simulink model "HeliDraft_26_02_2025"  (R2024b)
settings: Solver=VariableStepAuto  StartTime=0.0  StopTime=10.0  RelTol=1e-3
values from neighbouring files (symbols this model uses):
  R = D/2    (= 2.01773704722)    [untitled.m]
undefined symbols (not defined in the file or in its folder): Afin, AngVel, AngVeltr, BatteryCap, BatteryDischrgRate, Earth, EngPowSL, Ion, Lfin, Lithium, MTOW, Preq2RPM, RPM2Vreq, WGS84
libraries: fl_lib x7, nesl_utility x5, simulink_extras x4, aerolibatmos2 x2, aerolibanimutils x2, aerolibfltsims x2, aerolibtransform2 x1, shared6dof x1, batteryecm_lib x1, spsBatteryLib x1, spsControlledCurrentSourceLib x1, spspowerguiLib x1
(part 1 of 2)
settings Model: Creator=stand-alone1  LastModifiedBy=stand-alone1

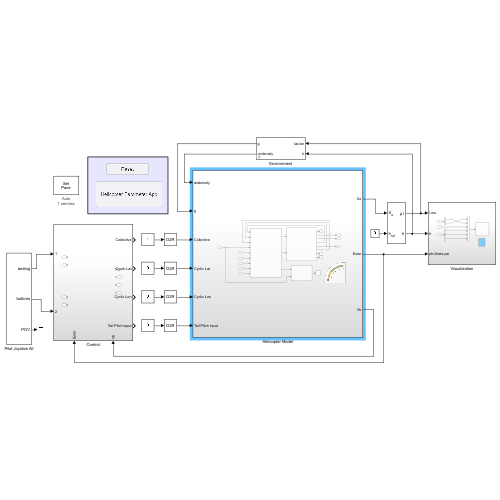
[thumbnail: Simulink's stored preview of the top-level diagram]
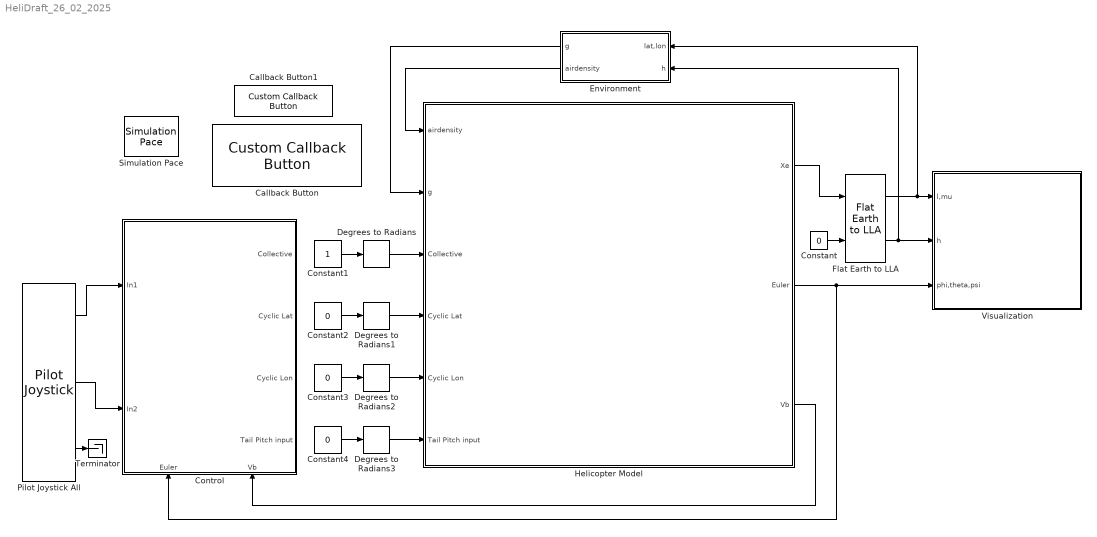
== system HeliDraft_26_02_2025 ==
  Callback Button : CustomCallbackButton  Configuration="{\"components\":[{\"name\":\"BackgroundImageComponent\",\"settings\":{\"image\":{\"size\":[0,0],\"src\":\"default\",\"srcOrientation\":\"Right\"},\"position\":[0,0,1,1]}},{\"name\":\"ButtonStateComponent\",\"settings\":{\"buttonType\":\"momentary\",\"clickFcn\":\"run(\\\"HelicopterParameterEstimation.mlapp\\\");\",\"onValue\":1,\"position\":[0,0,1,1],\"pressDelay\":\"500\",\"pressFcn\":\"\",\"repeatInterval\":\"0\",\"states\":[{\"horizontalAlignment\":\"center\",\"image\":{\"position\":[0,0,1,1],\"size\":[1,1],\"src\":\"default\",\"srcOrientation\":\"Right\"},\"label\":{\"color\":[0.01176470588,0.01176470588,0.01176470588,1],\"icon\":{\"size\":[0,0],\"src\":\"default\",\"srcOrientation\":\"Right\"},\"iconOffset\":0,\"iconPlacement\":\"left\",\"opacity\":1,\"show\":true,\"text\":{\"content\":\"Helicopter Parameter App\",\"font\":\"Helvetica\"}},\"labelOffset\":[0,0],\"verticalAlignment\":\"middle\"},{\"horizontalAlignment\":\"center\",\"image\":{\"position\":[0,0,1,1],\"size\":[1,1],\"src\":\"default\",\"srcOrientation\":\"Right\"},\"label\":{\"color\":[0.01176470588,0.01176470588,0.01176470588,1],\"icon\":{\"size\":[0,0],\"src\":\"default\",\"srcOrientation\":\"Right\"},\"iconOffset\":0,\"iconPlacement\":\"left\",\"opacity\":1,\"show\":true,\"text\":{\"content\":\"Helicopter Parameter App\",\"font\":\"Helvetica\"}},\"labelOffset\":[0,0],\"verticalAlignment\":\"middle\"},{\"horizontalAlignment\":\"center\",\"image\":{\"position\":[0,0,1,1],\"size\":[1,1],\"src\":\"default\",\"srcOrientation\":\"Right\"},\"label\":{\"color\":[0.01176470588,0.01176470588,0.01176470588,1],\"icon\":{\"size\":[0,0],\"src\":\"default\",\"srcOrientation\":\"Right\"},\"iconOffset\":0,\"iconPlacement\":\"left\",\"opacity\":1,\"show\":true,\"text\":{\"content\":\"Helicopter Parameter App\",\"font\":\"Helvetica\"}},\"labelOffset\":[0,0],\"verticalAlignment\":\"middle\"},{\"horizontalAlignment\":\"center\",\"image\":{\"position\":[0,0,1,1],\"size\":[1,1],\"src\":\"default\",\"srcOrientation\":\"Right\"},\"label\":{\"color\":[0.01176470588,0.01176470588,0.01176470588,1],\"icon\":{\"size\":[0,0],\"src\":\"default\",\"srcOrientation\":\"Right\"},\"iconOffset\":0,\"iconPlacement\":\"left\",\"opacity\":1,\"show\":true,\"text\":{\"content\":\"Helicopter Parameter App\",\"font\":\"Helvetica\"}},\"labelOffset\":[0,0],\"verticalAlignment\":\"middle\"}]}},{\"name\":\"ForegroundImageComponent\",\"settings\":{\"image\":{\"size\":[0,0],\"src\":\"default\",\"srcOrientation\":\"Right\"},\"isForeground\":1,\"position\":[0,0,1,1]}}],\"settings\":{\"BindingType\":\"standalone\",\"backgroundColor\":[244,244,244,1],\"backgroundOffset\":0.2,\"backgroundOpacity\":1,\"fixedAspectRatio\":\"off\",\"foregroundColor\":[0.01176470588,0.01176470588,0.01176470588,1],\"migratedFromLegacy\":true,\"useBackgroundColor\":true,\"variant\":\"callback\",\"version\":\"R2023a\"},\"type\":\"Button\"}"  CustomBackgroundColor="{\"color\":[0.9568627451,0.9568627451,0.9568627451],\"show\":true}"
  Callback Button1 : CustomCallbackButton  Configuration="{\"components\":[{\"name\":\"BackgroundImageComponent\",\"settings\":{\"image\":{\"size\":[0,0],\"src\":\"default\",\"srcOrientation\":\"Right\"},\"position\":[0,0,1,1]}},{\"name\":\"ButtonStateComponent\",\"settings\":{\"buttonType\":\"momentary\",\"clickFcn\":\"clc; clear; close all;\",\"onValue\":1,\"position\":[0,0,1,1],\"pressDelay\":\"500\",\"pressFcn\":\"\",\"repeatInterval\":\"0\",\"states\":[{\"horizontalAlignment\":\"center\",\"image\":{\"position\":[0,0,1,1],\"size\":[1,1],\"src\":\"default\",\"srcOrientation\":\"Right\"},\"label\":{\"color\":[0.01176470588,0.01176470588,0.01176470588,1],\"icon\":{\"size\":[0,0],\"src\":\"default\",\"srcOrientation\":\"Right\"},\"iconOffset\":0,\"iconPlacement\":\"left\",\"opacity\":1,\"show\":true,\"text\":{\"content\":\"Reset\",\"font\":\"Helvetica\"}},\"labelOffset\":[0,0],\"verticalAlignment\":\"middle\"},{\"horizontalAlignment\":\"center\",\"image\":{\"position\":[0,0,1,1],\"size\":[1,1],\"src\":\"default\",\"srcOrientation\":\"Right\"},\"label\":{\"color\":[0.01176470588,0.01176470588,0.01176470588,1],\"icon\":{\"size\":[0,0],\"src\":\"default\",\"srcOrientation\":\"Right\"},\"iconOffset\":0,\"iconPlacement\":\"left\",\"opacity\":1,\"show\":true,\"text\":{\"content\":\"Reset\",\"font\":\"Helvetica\"}},\"labelOffset\":[0,0],\"verticalAlignment\":\"middle\"},{\"horizontalAlignment\":\"center\",\"image\":{\"position\":[0,0,1,1],\"size\":[1,1],\"src\":\"default\",\"srcOrientation\":\"Right\"},\"label\":{\"color\":[0.01176470588,0.01176470588,0.01176470588,1],\"icon\":{\"size\":[0,0],\"src\":\"default\",\"srcOrientation\":\"Right\"},\"iconOffset\":0,\"iconPlacement\":\"left\",\"opacity\":1,\"show\":true,\"text\":{\"content\":\"Reset\",\"font\":\"Helvetica\"}},\"labelOffset\":[0,0],\"verticalAlignment\":\"middle\"},{\"horizontalAlignment\":\"center\",\"image\":{\"position\":[0,0,1,1],\"size\":[1,1],\"src\":\"default\",\"srcOrientation\":\"Right\"},\"label\":{\"color\":[0.01176470588,0.01176470588,0.01176470588,1],\"icon\":{\"size\":[0,0],\"src\":\"default\",\"srcOrientation\":\"Right\"},\"iconOffset\":0,\"iconPlacement\":\"left\",\"opacity\":1,\"show\":true,\"text\":{\"content\":\"Reset\",\"font\":\"Helvetica\"}},\"labelOffset\":[0,0],\"verticalAlignment\":\"middle\"}]}},{\"name\":\"ForegroundImageComponent\",\"settings\":{\"image\":{\"size\":[0,0],\"src\":\"default\",\"srcOrientation\":\"Right\"},\"isForeground\":1,\"position\":[0,0,1,1]}}],\"settings\":{\"BindingType\":\"standalone\",\"backgroundColor\":[244,244,244,1],\"backgroundOffset\":0.2,\"backgroundOpacity\":1,\"fixedAspectRatio\":\"off\",\"foregroundColor\":[0.01176470588,0.01176470588,0.01176470588,1],\"migratedFromLegacy\":true,\"useBackgroundColor\":true,\"variant\":\"callback\",\"version\":\"R2023a\"},\"type\":\"Button\"}"  CustomBackgroundColor="{\"color\":[0.9568627451,0.9568627451,0.9568627451],\"show\":true}"
  Constant{,2..4} (4 alike) : Constant  Value=0
  Constant1 : Constant
  Control : Subsystem
      settings: PortSchema="{\"entries\":[{\"content\":{\"sides\":[{\"content\":{\"connectorIds\":[\"In1\",\"In2\"]},\"type\":\"ConnectorPlacement.EquallySpacedRectSide\",\"uuid\":\"528401e7-0fef-44be-ba63-acf96d247fb7\"},{\"content\":{\"connectorIds\":[\"Out1\",\"Out2\",\"Out3\",\"Out4\"],\"side\":\"RIGHT\"},\"type\":\"ConnectorPlacement.EquallySpacedRectSide\",\"uuid\":\"314663aa-6cd9-4175-a49a-1575f8a7b87b\"},{\"content\":{\"side\":\"TOP\"},\"type\":\"ConnectorPlacement.EquallySpacedRectSide\",\"uuid\":\"d6c3b2b9-365b-49fe-86cc-8f0c15878230\"},{\"content\":{\"connectorIds\":[\"In3\",\"In4\"],\"side\":\"BOTTOM\"},\"type\":\"ConnectorPlacement.EquallySpacedRectSide\",\"uuid\":\"be77d0ba-d3ca-47ac-ab5e-0cf95d8527f7\"}]},\"type\":\"ConnectorPlacement.EquallySpacedConnector\",\"uuid\":\"719848b2-01be-4853-b472-0e21e9b8be5c\"}],\"packageUris\":[\"http://schema.mathworks.com/mf0/Connector/R2020b\"],\"version\":\"1.0\"}"
  Degrees to Radians{,1..3} (4 alike) : simulink_extras/Transformations/Degrees to Radians
  Environment : Subsystem  mask{atmomodel=ISA, consg=on, Parameter3=on}
      mask prompts: atmomodel "Atmosphere Model"; consg "Constant g (Gravitational Acceleration)"; Parameter3 "On/Off"
      mask DialogControl a Prompt: Environment
      mask DialogControl b Prompt: Wind simulation, atmosphere properties and gravity model
      mask DialogControl Container4 Prompt: Environment
      mask DialogControl Container5 Prompt: Wind
  Flat Earth to LLA : aerolibtransform2/Flat Earth to LLA  units=Metric (MKS)  ptype=Earth (WGS84)  F=1/298.257223563  R=6378137  refPosPort=off  LL0=[0 10]  psi=0
  Helicopter Model : Subsystem
  Pilot Joystick All : aerolibanimutils/Pilot Joystick  JoystickID=Joystick1  OutputConfiguration=AllOutputs  SampleTime=1/30
      settings: LibrarySourceBlock=aerolibanimutils/Pilot Joystick All
  Simulation Pace : aerolibanimutils/Simulation Pace  SimulationPace=1  SleepMode=Auto  OutputPaceError=off  SampleTime=1/30
  Terminator : Terminator
  Visualization : Subsystem
  wires:
  Constant/1 -> Flat Earth to LLA/2
  Flat Earth to LLA/1 -> Environment/1(lat,lon), Visualization/1(l,mu)
  Flat Earth to LLA/2 -> Environment/2(h), Visualization/2(h)
  Pilot Joystick All/1 -> Control/1(In1)
  Pilot Joystick All/2 -> Control/2(In2)
  Environment/1(g) -> Helicopter Model/2(g)
  Environment/2(airdensity) -> Helicopter Model/1(airdensity)
  Helicopter Model/1(Xe) -> Flat Earth to LLA/1
  Helicopter Model/2(Euler) -> Visualization/3(phi,theta,psi), Control/3(Euler)
  Pilot Joystick All/3 -> Terminator/1
  Helicopter Model/3(Vb) -> Control/4(Vb)
  Constant1/1 -> Degrees to Radians/1
  Constant2/1 -> Degrees to Radians1/1
  Constant3/1 -> Degrees to Radians2/1
  Constant4/1 -> Degrees to Radians3/1
  Degrees to Radians/1 -> Helicopter Model/3(Collective)
  Degrees to Radians1/1 -> Helicopter Model/4(Cyclic Lat)
  Degrees to Radians2/1 -> Helicopter Model/5(Cyclic Lon)
  Degrees to Radians3/1 -> Helicopter Model/6(Tail Pitch input)

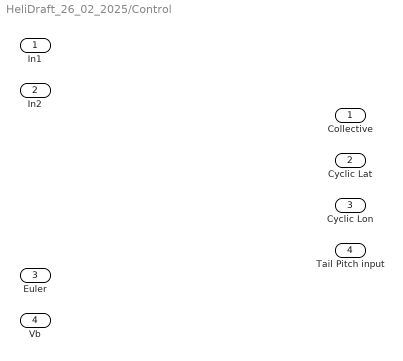
== system HeliDraft_26_02_2025/Control ==
  In1 : Inport
  In2 : Inport  Port=2
  Euler : Inport  Port=3
  Vb : Inport  Port=4
  Collective : Outport
  Cyclic Lat : Outport  Port=2
  Cyclic Lon : Outport  Port=3
  Tail Pitch input : Outport  Port=4

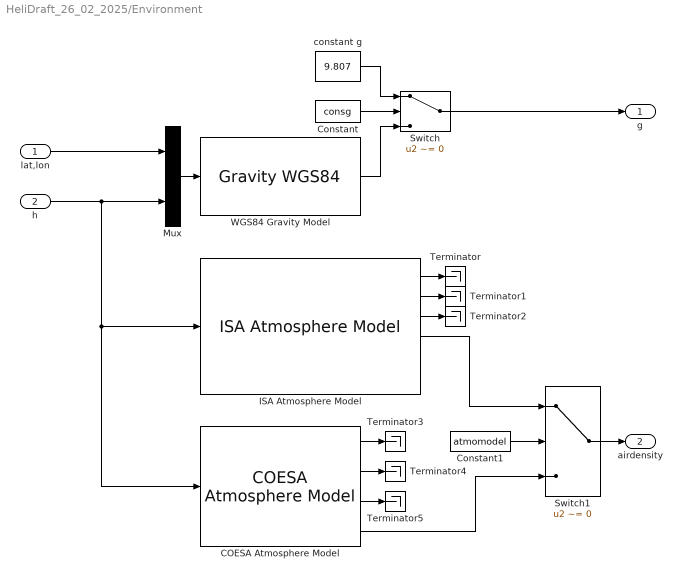
== system HeliDraft_26_02_2025/Environment ==
  lat,lon : Inport
  h : Inport  Port=2
  COESA Atmosphere Model : aerolibatmos2/COESA Atmosphere Model  units=Metric (MKS)  spec=1976 COESA-extended U.S. Standard Atmosphere  model=Profile  profile_var=High temperature  profile_percent=1%  profile_alt=5 km (16404 ft)  envelope_var=High temperature  envelope_percent=1%  action=Warning
  Constant : Constant  Value=consg
  Constant1 : Constant  Value=atmomodel
  ISA Atmosphere Model : aerolibatmos2/ISA Atmosphere Model  useExtended=off  action=Warning  custom=off  viscosityOut=on  g=9.80665  gamma=1.4  R=287.0531  L=0.0065  h_trop=11000  h_strat=20000  rho0=1.225  P0=101325  T0=288.15  h0=0  S=110.4  Tref=273.15  muref=1.716e-5
  Mux : Mux  Inputs=2
  Switch : Switch  Criteria=u2 ~= 0  SaturateOnIntegerOverflow=off  InputSameDT=off
  Switch1 : Switch  Criteria=u2 ~= 0  SaturateOnIntegerOverflow=off  InputSameDT=off
  Terminator{,1..5} (6 alike) : Terminator
  "WGS84 Gravity Model  " : GravityWGS84
  constant g : Constant  Value=9.807
  g : Outport
  airdensity : Outport  Port=2
  wires:
  lat,lon/1 -> Mux/1
  Constant/1 -> Switch/2
  constant g/1 -> Switch/1
  "WGS84 Gravity Model  "/1 -> Switch/3
  Switch/1 -> g/1
  Mux/1 -> "WGS84 Gravity Model  "/1
  h/1 -> COESA Atmosphere Model/1, ISA Atmosphere Model/1, Mux/2
  Switch1/1 -> airdensity/1
  ISA Atmosphere Model/1 -> Terminator/1
  ISA Atmosphere Model/2 -> Terminator1/1
  ISA Atmosphere Model/3 -> Terminator2/1
  COESA Atmosphere Model/2 -> Terminator4/1
  COESA Atmosphere Model/1 -> Terminator3/1
  COESA Atmosphere Model/3 -> Terminator5/1
  ISA Atmosphere Model/4 -> Switch1/1
  COESA Atmosphere Model/4 -> Switch1/3
  Constant1/1 -> Switch1/2

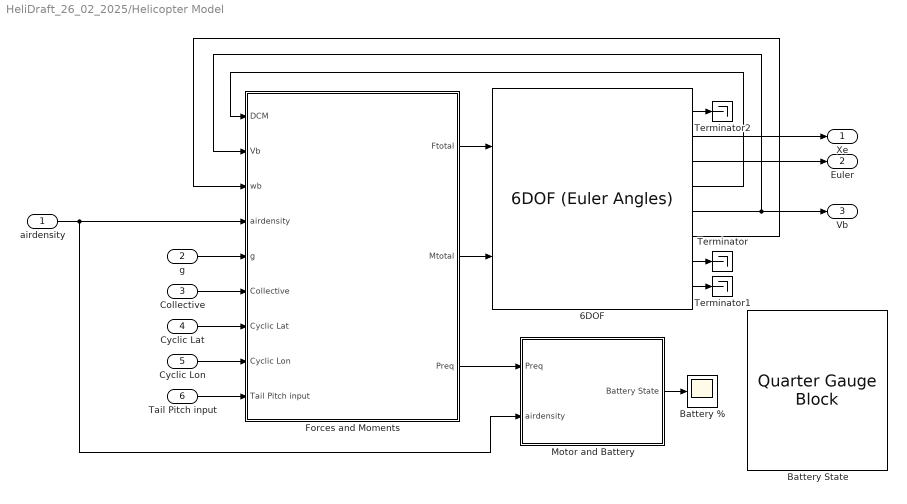
== system HeliDraft_26_02_2025/Helicopter Model ==
  airdensity : Inport
  g : Inport  Port=2
  Collective : Inport  Port=3
  Cyclic Lat : Inport  Port=4
  Cyclic Lon : Inport  Port=5
  Tail Pitch input : Inport  Port=6
  6DOF : shared6dof/6DOF (Euler Angles)  units=Metric (MKS)  mtype=Fixed  rep=Euler Angles  xme_0=[0 0 0]  Vm_0=[0 0 0]  eul_0=[0 0 0]  pm_0=[0 0 0]  mass_0=MTOW  mass_e=0.5  mass_f=2.0  inertia=eye(3)  inertia_e=eye(3)  inertia_f=2*eye(3)  k_quat=1.0  vre_flag=off  abi_flag=off  aMode=0  xme_statename=''  Vm_statename=''  eul_statename=''  quat_statename=''  pm_statename=''  mass_statename=''
  Battery % : Scope
  Battery State : QuarterGaugeBlock  LabelPosition=Hide
  Forces and Moments : Subsystem
  Motor and Battery : Subsystem
  Terminator : Terminator
  Terminator1 : Terminator
  Terminator2 : Terminator
  Xe : Outport
  Euler : Outport  Port=2
  Vb : Outport  Port=3
  wires:
  6DOF/1 -> Terminator2/1
  6DOF/8 -> Terminator1/1
  Forces and Moments/1(Ftotal) -> 6DOF/1
  Forces and Moments/2(Mtotal) -> 6DOF/2
  6DOF/6 -> Forces and Moments/3(wb)
  6DOF/4 -> Forces and Moments/1(DCM)
  6DOF/7 -> Terminator/1
  6DOF/5 -> Vb/1, Forces and Moments/2(Vb)
  Cyclic Lat/1 -> Forces and Moments/7(Cyclic Lat)
  Collective/1 -> Forces and Moments/6(Collective)
  6DOF/3 -> Euler/1
  Tail Pitch input/1 -> Forces and Moments/9(Tail Pitch input)
  Cyclic Lon/1 -> Forces and Moments/8(Cyclic Lon)
  airdensity/1 -> Forces and Moments/4(airdensity), Motor and Battery/2(airdensity)
  g/1 -> Forces and Moments/5(g)
  6DOF/2 -> Xe/1
  Forces and Moments/3(Preq) -> Motor and Battery/1(Preq)
  Motor and Battery/1(Battery State) -> Battery %/1

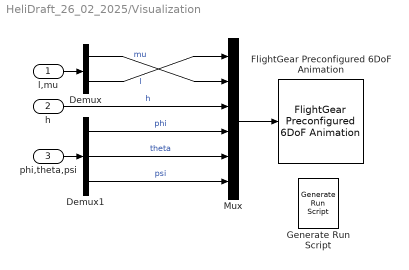
== system HeliDraft_26_02_2025/Visualization ==
  l,mu : Inport
  h : Inport  Port=2
  phi,theta,psi : Inport  Port=3
  Demux : Demux  Outputs=2
  Demux1 : Demux  Outputs=3
  "FlightGear Preconfigured 6DoF Animation " : aerolibfltsims/FlightGear Preconfigured 6DoF Animation  xFlightGearVersion=v2019.1  DestinationIpAddress=127.0.0.1  DestinationPort=5502  SampleTime=1/30  packetVersion=24
  "Generate Run Script " : aerolibfltsims/Generate Run Script  Architecture=Default  dataFlow=Send  GeometryModelName=HL20  AirportId=KSFO  RunwayId=10L  InitialAltitude=7224  InitialHeading=113  OffsetDistance=4.72  OffsetAzimuth=0  InstallScenery=off  DisableShaders=off  OriginAddress=127.0.0.1  DestinationPort=5502  OriginPort=5505  LocalAddress=127.0.0.1  OutputFileName=runfg.bat  FlightGearBaseDirectory=C:\Program Files\FlightGear
  Mux : Mux  Inputs=6
  wires:
  l,mu/1 -> Demux/1
  Demux/2 -> Mux/1  "l"
  Demux/1 -> Mux/2  "mu"
  Mux/1 -> "FlightGear Preconfigured 6DoF Animation "/1
  h/1 -> Mux/3  "h"
  Demux1/1 -> Mux/4  "phi"
  Demux1/2 -> Mux/5  "theta"
  Demux1/3 -> Mux/6  "psi"
  phi,theta,psi/1 -> Demux1/1

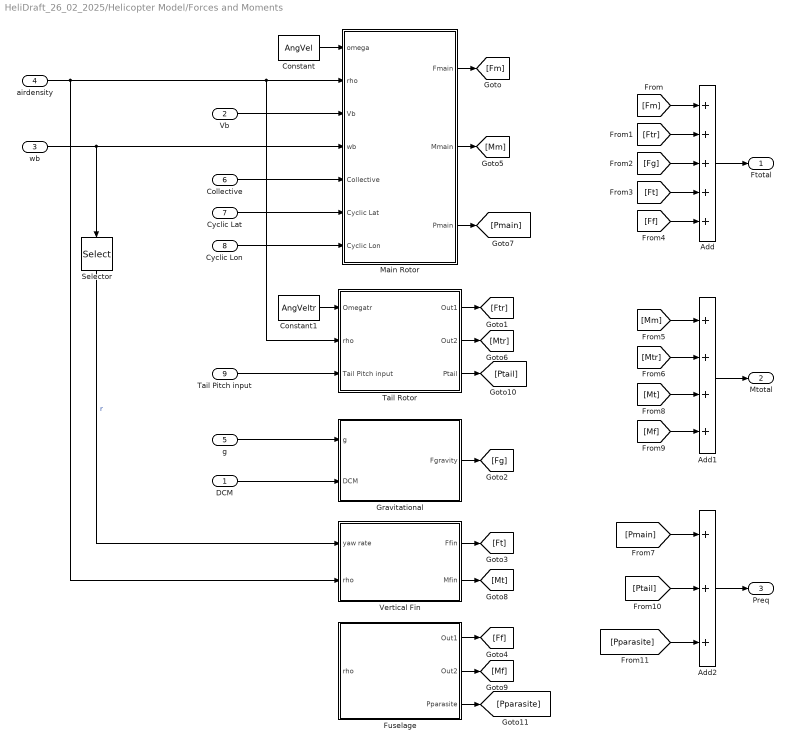
== system HeliDraft_26_02_2025/Helicopter Model/Forces and Moments ==
  DCM : Inport
  Vb : Inport  Port=2
  wb : Inport  Port=3
  airdensity : Inport  Port=4
  g : Inport  Port=5
  Collective : Inport  Port=6
  Cyclic Lat : Inport  Port=7
  Cyclic Lon : Inport  Port=8
  Tail Pitch input : Inport  Port=9
  Add : Sum  Inputs=+++++
  Add1 : Sum  Inputs=++++
  Add2 : Sum  Inputs=+++
  Constant : Constant  Value=AngVel
  Constant1 : Constant  Value=AngVeltr
  Fuselage : Subsystem
  Gravitational : Subsystem
  Main Rotor : Subsystem
  Selector : Selector  InputPortWidth=3  IndexOptions=Index vector (dialog)  Indices=[3]  OutputSizes=1
  Tail Rotor : Subsystem
  Vertical Fin : Subsystem
  Ftotal : Outport
  Mtotal : Outport  Port=2
  Preq : Outport  Port=3
  wires:
  Add/1 -> Ftotal/1
  Add1/1 -> Mtotal/1
  Main Rotor/1(Fmain) -> [Fm]
  Tail Rotor/1(Out1) -> [Ftr]
  Gravitational/1(Fgravity) -> [Fg]
  Vertical Fin/1(Ffin) -> [Ft]
  Fuselage/1(Out1) -> [Ff]
  [Fm] -> Add/1
  [Ftr] -> Add/2
  [Fg] -> Add/3
  [Ft] -> Add/4
  [Ff] -> Add/5
  Main Rotor/2(Mmain) -> [Mm]
  Tail Rotor/2(Out2) -> [Mtr]
  Vertical Fin/2(Mfin) -> [Mt]
  Fuselage/2(Out2) -> [Mf]
  [Mm] -> Add1/1
  [Mtr] -> Add1/2
  [Mf] -> Add1/4
  [Mt] -> Add1/3
  Constant/1 -> Main Rotor/1(omega)
  Constant1/1 -> Tail Rotor/1(Omegatr)
  airdensity/1 -> Vertical Fin/2(rho), Tail Rotor/2(rho), Main Rotor/2(rho)
  g/1 -> Gravitational/1(g)
  DCM/1 -> Gravitational/2(DCM)
  Collective/1 -> Main Rotor/5(Collective)
  Tail Pitch input/1 -> Tail Rotor/3(Tail Pitch input)
  Cyclic Lat/1 -> Main Rotor/6(Cyclic Lat)
  Cyclic Lon/1 -> Main Rotor/7(Cyclic Lon)
  wb/1 -> Selector/1, Main Rotor/4(wb)
  Vb/1 -> Main Rotor/3(Vb)
  Add2/1 -> Preq/1
  Main Rotor/3(Pmain) -> [Pmain]
  Tail Rotor/3(Ptail) -> [Ptail]
  Fuselage/3(Pparasite) -> [Pparasite]
  [Pmain] -> Add2/1
  [Ptail] -> Add2/2
  [Pparasite] -> Add2/3
  Selector/1 -> Vertical Fin/1(yaw rate)  "r"

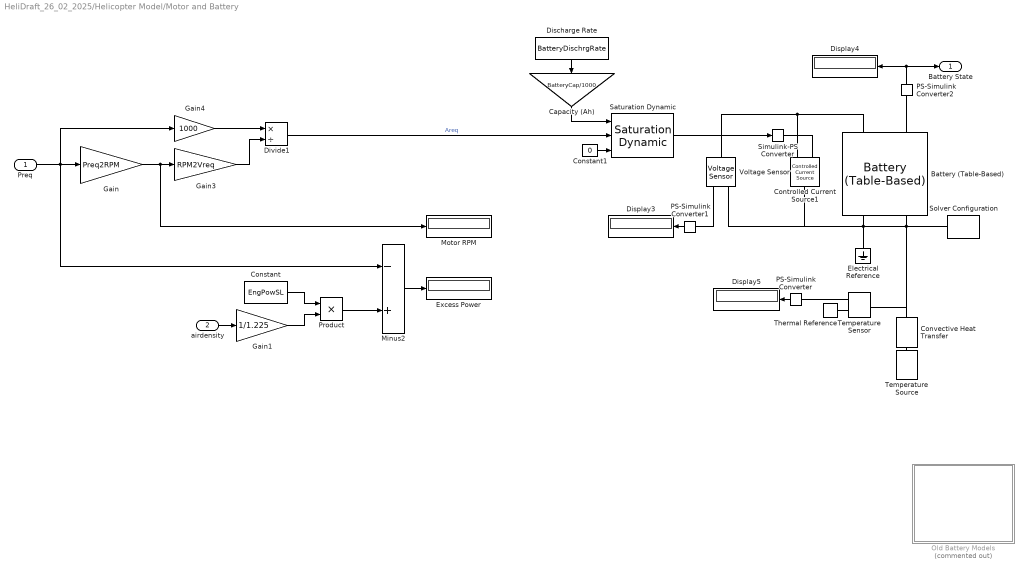
== system HeliDraft_26_02_2025/Helicopter Model/Motor and Battery ==
  Preq : Inport
  airdensity : Inport  Port=2
  Battery (Table-Based) : batteryecm_lib/Battery (Table-Based)  PartSpecification="{\"DatasetId\":\"Valence|U27_36XP|simscape.battery.batteryTableBased\",\"DisplayName\":\"Valence:U27_36XP\"}"  SOC_vec=[0 0.01 0.02 0.03 0.04 0.05 0.06 0.07 0.08 0.09 0.1 0.11 0.12 0.13 0.14 0.15 0.16 0.17 0.18 0.19 0.2 0.21 0.22 0.23 0.24 0.25 0.26 0.27 0.28 0.29 0.3 0.31 0.32 0.33 0.34 0.35 0.36 0.37 0.38 0.39 0.4 0.41 0.42 0.43 0.44 0.45 0.46 0.47 0.48 0.49 0.5 0.51 0.52 0.53 0.54 0.55 0.56 0.57 0.58 0.59 0.6 0.61 0.62 0.63 0.64 0.65 0.66 0.67 0.68 0.69 0.7 0.71 0.72 0.73 0.74 0.75 0.76 0.77 0.78 0.79 0.8 0.81 0.82 0.83 0.84 0.85 0.86 0.87 0.88 0.89 0.9 0.91 0.92 0.93 0.94 0.95 0.96 0.97 0.98 0.99 1] % Datasheet derived  T_dependence=simscape.enum.tablebattery.temperature_dependence.yes  prm_dir=simscape.enum.tablebattery.prm_dir.noCurrentDirectionality  T_vec=[-10 0 10 20 23 30 40 50] % Datasheet derived degC  V0_mat=[35.84591 35.84591 35.84591 35.84591 35.84591 35.84591 35.84591 35.84591;36.10202 36.10202 36.10202 36.10202 36.10202 36.10202 36.10202 36.10202;36.35814 36.35814 36.35814 36.35814 36.35814 36.35814 36.35814 36.35814;36.61425 36.61425 36.61425 36.61425 36.61425 36.61425 36.61425 36.61425;36.87037 36.87037 36.87037 36.87037 36.87037 36.87037 36.87037 36.87037;37.12649 37.12649 37.12649 37.12649 37.12649 37.12649 37.12649 37.12649;37.3826 37.3826 37.3826 37.3826 37.3826 37.3826 37.3826 37.3826;37.63872 37.63872 37.63872 37.63872 37.63872 37.63872 37.63872 37.63872;37.89483 37.89483 37.89483 37.89483 37.89483 37.89483 37.89483 37.89483;38.09951 38.09951 38.09951 38.09951 38.09951 38.09951 38.09951 38.09951;38.20904 38.20904 38.20904 38.20904 38.20904 38.20904 38.20904 38.20904;38.28916 38.28916 38.28916 38.28916 38.28916 38.28916 38.28916 38.28916;38.37306 38.37306 38.37306 38.37306 38.37306 38.37306 38.37306 38.37306;38.42308 38.42308 38.42308 38.42308 38.42308 38.42308 38.42308 38.42308;38.45482 38.45482 38.45482 38.45482 38.45482 38.45482 38.45482 38.45482;38.47744 38.47744 38.47744 38.47744 38.47744 38.47744 38.47744 38.47744;38.49779 38.49779 38.49779 38.49779 38.49779 38.49779 38.49779 38.49779;38.54815 38.54815 38.54815 38.54815 38.54815 38.54815 38.54815 38.54815;38.5883 38.5883 38.5883 38.5883 38.5883 38.5883 38.5883 38.5883;38.63829 38.63829 38.63829 38.63829 38.63829 38.63829 38.63829 38.63829;38.68732 38.68732 38.68732 38.68732 38.68732 38.68732 38.68732 38.68732;38.72975 38.72975 38.72975 38.72975 38.72975 38.72975 38.72975 38.72975;38.77111 38.77111 38.77111 38.77111 38.77111 38.77111 38.77111 38.77111;38.80795 38.80795 38.80795 38.80795 38.80795 38.80795 38.80795 38.80795;38.83724 38.83724 38.83724 38.83724 38.83724 38.83724 38.83724 38.83724;38.8617 38.8617 38.8617 38.8617 38.8617 38.8617 38.8617 38.8617;38.89023 38.89023 38.89023 38.89023 38.89023 38.89023 38.89023 38.89023;38.9273 38.9273 38.9273 38.9273 38.9273 38.9273 38.9273 38.9273;38.96054 38.96054 38.96054 38.96054 38.96054 38.96054 38.96054 38.96054;38.98786 38.98786 38.98786 38.98786 38.98786 38.98786 38.98786 38.98786;39.01519 39.01519 39.01519 39.01519 39.01519 39.01519 39.01519 39.01519;39.03864 39.03864 39.03864 39.03864 39.03864 39.03864 39.03864 39.03864;39.06385 39.06385 39.06385 39.06385 39.06385 39.06385 39.06385 39.06385;39.08223 39.08223 39.08223 39.08223 39.08223 39.08223 39.08223 39.08223;39.1006 39.1006 39.1006 39.1006 39.1006 39.1006 39.1006 39.1006;39.11898 39.11898 39.11898 39.11898 39.11898 39.11898 39.11898 39.11898;39.13735 39.13735 39.13735 39.13735 39.13735 39.13735 39.13735 39.13735;39.15508 39.15508 39.15508 39.15508 39.15508 39.15508 39.15508 39.15508;39.16412 39.16412 39.16412 39.16412 39.16412 39.16412 39.16412 39.16412;39.17437 39.17437 39.17437 39.17437 39.17437 39.17437 39.17437 39.17437;39.18528 39.18528 39.18528 39.18528 39.18528 39.18528 39.18528 39.18528;39.19619 39.19619 39.19619 39.19619 39.19619 39.19619 39.19619 39.19619;39.20709 39.20709 39.20709 39.20709 39.20709 39.20709 39.20709 39.20709;39.21696 39.21696 39.21696 39.21696 39.21696 39.21696 39.21696 39.21696;39.22232 39.22232 39.22232 39.22232 39.22232 39.22232 39.22232 39.22232;39.22753 39.22753 39.22753 39.22753 39.22753 39.22753 39.22753 39.22753;39.23277 39.23277 39.23277 39.23277 39.23277 39.23277 39.23277 39.23277;39.23672 39.23672 39.23672 39.23672 39.23672 39.23672 39.23672 39.23672;39.23942 39.23942 39.23942 39.23942 39.23942 39.23942 39.23942 39.23942;39.24211 39.24211 39.24211 39.24211 39.24211 39.24211 39.24211 39.24211;39.24481 39.24481 39.24481 39.24481 39.24481 39.24481 39.24481 39.24481;39.24786 39.24786 39.24786 39.24786 39.24786 39.24786 39.24786 39.24786;39.25094 39.25094 39.25094 39.25094 39.25094 39.25094 39.25094 39.25094;39.2539 39.2539 39.2539 39.2539 39.2539 39.2539 39.2539 39.2539;39.25686 39.25686 39.25686 39.25686 39.25686 39.25686 39.25686 39.25686;39.26099 39.26099 39.26099 39.26099 39.26099 39.26099 39.26099 39.26099;39.26708 ...(+3199 chars)] % Datasheet derived V  V0_vec=[35.84591 36.10202 36.35814 36.61425 36.87037 37.12649 37.3826 37.63872 37.89483 38.09951 38.20904 38.28916 38.37306 38.42308 38.45482 38.47744 38.49779 38.54815 38.5883 38.63829 38.68732 38.72975 38.77111 38.80795 38.83724 38.8617 38.89023 38.9273 38.96054 38.98786 39.01519 39.03864 39.06385 39.08223 39.1006 39.11898 39.13735 39.15508 39.16412 39.17437 39.18528 39.19619 39.20709 39.21696 39.22232 39.22753 39.23277 39.23672 39.23942 39.24211 39.24481 39.24786 39.25094 39.2539 39.25686 39.26099 39.26708 39.27551 39.28394 39.29233 39.30067 39.31557 39.33487 39.35402 39.37113 39.38825 39.40815 39.43406 39.46187 39.48968 39.51913 39.55031 39.5817 39.60619 39.62271 39.63907 39.65521 39.67134 39.68137 39.69071 39.70005 39.7052 39.70868 39.70916 39.70862 39.70807 39.70752 39.71037 39.72142 39.72908 39.73651 39.73911 39.73577 39.72919 39.73278 39.7392 39.74638 39.75462 39.8136 40.01141 40.30627] % Datasheet derived V  V_range=[27 Inf] % Datasheet derived V  R0_mat=[0.9112 0.73319 0.55116 0.3909 0.47635 0.31145 0.24894 0.23351;0.9112 0.79214 0.50936 0.32708 0.41138 0.21289 0.15029 0.11642;0.9112 0.75838 0.46755 0.26325 0.35007 0.14203 0.09214 0.07324;0.9112 0.72463 0.42575 0.19942 0.29417 0.09634 0.05758 0.04021;0.9112 0.69087 0.38395 0.15149 0.24882 0.06764 0.03364 0.02182;0.9112 0.65711 0.34215 0.11725 0.2142 0.04885 0.01957 0.00983;0.9112 0.62335 0.30035 0.09581 0.18886 0.03484 0.01134 0.00372;0.88245 0.58959 0.25855 0.08105 0.17031 0.02886 0.01013 0.00445;0.85369 0.55583 0.22327 0.07125 0.1569 0.02915 0.01483 0.00976;0.82493 0.52207 0.19506 0.06386 0.14398 0.03152 0.0196 0.01392;0.79618 0.48831 0.16793 0.05824 0.13028 0.031 0.02172 0.01735;0.76742 0.45455 0.14437 0.05231 0.11716 0.03152 0.02306 0.0196;0.73866 0.42079 0.12447 0.04884 0.10632 0.03219 0.02454 0.02192;0.70991 0.38703 0.1096 0.04638 0.09512 0.03151 0.02458 0.0216;0.68115 0.35327 0.09525 0.04318 0.08414 0.02987 0.02387 0.02054;0.65239 0.31952 0.08121 0.03996 0.07347 0.02787 0.02226 0.01912;0.62364 0.27915 0.07388 0.03692 0.06467 0.02578 0.02045 0.01757;0.59488 0.24506 0.06774 0.03508 0.05964 0.02492 0.01984 0.01722;0.56612 0.21466 0.06284 0.03384 0.05477 0.02422 0.01882 0.01646;0.53737 0.18917 0.06009 0.03346 0.05154 0.02391 0.0187 0.0161;0.50861 0.16681 0.05729 0.03301 0.04841 0.02357 0.0188 0.0157;0.47986 0.14646 0.05423 0.03228 0.04625 0.02296 0.01864 0.01586;0.4511 0.13143 0.05231 0.0315 0.04448 0.02305 0.01844 0.01609;0.42234 0.11995 0.05123 0.03055 0.04297 0.02298 0.01851 0.01613;0.39359 0.10903 0.04985 0.03032 0.04112 0.02261 0.01828 0.01587;0.36483 0.09944 0.04828 0.02989 0.03908 0.02204 0.01786 0.01541;0.33607 0.09353 0.04687 0.02963 0.0378 0.02164 0.01762 0.01512;0.30291 0.08834 0.04648 0.02972 0.03771 0.02158 0.01779 0.01527;0.27067 0.08411 0.04619 0.02964 0.03746 0.0219 0.0178 0.01525;0.24264 0.08054 0.04566 0.02987 0.03699 0.02206 0.01758 0.015;0.21621 0.07803 0.04513 0.03012 0.03652 0.02222 0.01736 0.01476;0.19063 0.07544 0.04456 0.03022 0.03598 0.02223 0.01698 0.01435;0.17492 0.07417 0.04451 0.03039 0.03587 0.0223 0.01675 0.01402;0.15924 0.07263 0.04418 0.03029 0.03552 0.0221 0.01669 0.01376;0.14506 0.07109 0.04385 0.03019 0.03517 0.0219 0.01663 0.01361;0.13357 0.06955 0.04352 0.03009 0.03481 0.0217 0.01658 0.01346;0.12461 0.0686 0.04319 0.02998 0.03446 0.0215 0.01652 0.01331;0.11872 0.06771 0.04286 0.02995 0.03417 0.02128 0.01643 0.01313;0.11354 0.06648 0.04251 0.02967 0.03358 0.02084 0.016 0.01261;0.10849 0.0653 0.0422 0.02943 0.03336 0.02078 0.01562 0.01213;0.10559 0.06415 0.04193 0.02923 0.03321 0.02075 0.01526 0.01187;0.10269 0.06364 0.04165 0.02902 0.03305 0.02071 0.01515 0.01197;0.09978 0.06339 0.04137 0.02881 0.0329 0.02068 0.01521 0.01208;0.09733 0.06309 0.04105 0.02856 0.0327 0.0206 0.01523 0.01214;0.09518 0.06261 0.0406 0.02813 0.03227 0.02035 0.01507 0.01203;0.09303 0.06213 0.04031 0.0277 0.03186 0.02009 0.01491 0.01191;0.0912 0.06165 0.04003 0.02736 0.03148 0.01983 0.01474 0.01179;0.08999 0.06112 0.0397 0.02706 0.03105 0.01963 0.01452 0.01161;0.08874 0.06053 0.03932 0.02671 0.03058 0.0194 0.01426 0.01139;0.08749 0.05993 0.03893 0.02636 0.03011 0.01916 0.01399 0.01119;0.08652 0.05934 0.03855 0.02601 0.02964 0.01893 0.01372 0.01104;0.08605 0.05876 0.03818 0.02568 0.02918 0.01872 0.01346 0.01091;0.08557 0.05819 0.03788 0.02534 0.02875 0.0185 0.0132 0.01078;0.0851 0.0576 0.03759 0.025 0.02834 0.01828 0.01294 0.01065;0.08479 0.05702 0.0373 0.02466 0.02792 0.01806 0.01268 0.01051;0.08459 0.05663 0.03706 0.0244 0.02762 0.01789 0.01247 0.01042;0.08446 0.0566 0.0369 0.02423 0.02745 0.01779 0.01233 0.01038;0.08442 0.05667 0.03684 0.02414 0.02737 0.01779 0.01229 0.01018;0.08439 0.05674 0.03677 0.02406 0.02729 0.01777 0.01225 0.00997;0.08436 0.05681 0.0367 0.02397 0.02722 0.01767 0.01221 0.00977;0.08463 0.05687 0.03669 0.02389 0.02715 0.01757 0.01218 0.00956;0.08516 0.0572 0.03698 0.02406 0.0274 0.01773 0.0124 0.00962;0.08586 0.0577 0.03744 0.02442 0.02786 0.01806 0.0128 0.00985;0.08657 0.05819 0.0379 ...(+2382 chars)] % Datasheet derived Ohm  R0_vec=[0.47635 0.41138 0.35007 0.29417 0.24882 0.2142 0.18886 0.17031 0.1569 0.14398 0.13028 0.11716 0.10632 0.09512 0.08414 0.07347 0.06467 0.05964 0.05477 0.05154 0.04841 0.04625 0.04448 0.04297 0.04112 0.03908 0.0378 0.03771 0.03746 0.03699 0.03652 0.03598 0.03587 0.03552 0.03517 0.03481 0.03446 0.03417 0.03358 0.03336 0.03321 0.03305 0.0329 0.0327 0.03227 0.03186 0.03148 0.03105 0.03058 0.03011 0.02964 0.02918 0.02875 0.02834 0.02792 0.02762 0.02745 0.02737 0.02729 0.02722 0.02715 0.0274 0.02786 0.0283 0.02854 0.02877 0.02906 0.02956 0.03013 0.0307 0.03135 0.03204 0.03271 0.03308 0.03307 0.03314 0.03323 0.03332 0.03312 0.03288 0.03264 0.03224 0.03172 0.03113 0.03057 0.03001 0.02945 0.02905 0.02924 0.0293 0.02938 0.02923 0.02879 0.02803 0.02792 0.02793 0.02786 0.02652 0.02587 0.02701 0.00941] % Datasheet derived Ohm  R0_dis_mat=[.0117, .0085, .009; .011, .0085, .009; .0114, .0087, .0092; .0107, .0082, .0088; .0107, .0083, .0091; .0113, .0085, .0089; .0116, .0085, .0089] % Parameter not set Ohm  R0_dis_vec=[.0085, .0085, .0087, .0082, .0083, .0085, .0085] % Parameter not set Ohm  R0_ch_mat=[.0117, .0085, .009; .011, .0085, .009; .0114, .0087, .0092; .0107, .0082, .0088; .0107, .0083, .0091; .0113, .0085, .0089; .0116, .0085, .0089] % Parameter not set Ohm  R0_ch_vec=[.0085, .0085, .0087, .0082, .0083, .0085, .0085] % Parameter not set Ohm  AH=50.41 % Datasheet derived hr*A  prm_leak=simscape.enum.tablebattery.prm_leak.disabled  Rleak_vec=[8000, 7000, 6000] % Parameter not set Ohm  Rleak=7e3 % Parameter not set Ohm  extrapolation_option=simscape.enum.extrapolation.nearest  SOC_port=simscape.enum.tablebattery.enable.yes  prm_dyn=simscape.enum.tablebattery.prm_dyn.off  R1_mat=[.0109, .0029, .0013; .0069, .0024, .0012; .0047, .0026, .0013; .0034, .0016, .001; .0033, .0023, .0014; .0033, .0018, .0011; .0028, .0017, .0011] % Parameter not set Ohm  R1_vec=[.0029, .0024, .0026, .0016, .0023, .0018, .0017] % Parameter not set Ohm  tau1_mat=[20, 36, 39; 31, 45, 39; 109, 105, 61; 36, 29, 26; 59, 77, 67; 40, 33, 29; 25, 39, 33] % Parameter not set s  tau1_vec=[36, 45, 105, 29, 77, 33, 39] % Parameter not set s  R2_mat=[.0109, .0029, .0013; .0069, .0024, .0012; .0047, .0026, .0013; .0034, .0016, .001; .0033, .0023, .0014; .0033, .0018, .0011; .0028, .0017, .0011] % Parameter not set Ohm  R2_vec=[.0029, .0024, .0026, .0016, .0023, .0018, .0017] % Parameter not set Ohm  tau2_mat=[20, 36, 39; 31, 45, 39; 109, 105, 61; 36, 29, 26; 59, 77, 67; 40, 33, 29; 25, 39, 33] % Parameter not set s  tau2_vec=[36, 45, 105, 29, 77, 33, 39] % Parameter not set s  R3_mat=[.0109, .0029, .0013; .0069, .0024, .0012; .0047, .0026, .0013; .0034, .0016, .001; .0033, .0023, .0014; .0033, .0018, .0011; .0028, .0017, .0011] % Parameter not set Ohm  R3_vec=[.0029, .0024, .0026, .0016, .0023, .0018, .0017] % Parameter not set Ohm  tau3_mat=[20, 36, 39; 31, 45, 39; 109, 105, 61; 36, 29, 26; 59, 77, 67; 40, 33, 29; 25, 39, 33] % Parameter not set s  tau3_vec=[36, 45, 105, 29, 77, 33, 39] % Parameter not set s  R4_mat=[.0109, .0029, .0013; .0069, .0024, .0012; .0047, .0026, .0013; .0034, .0016, .001; .0033, .0023, .0014; .0033, .0018, .0011; .0028, .0017, .0011] % Parameter not set Ohm  R4_vec=[.0029, .0024, .0026, .0016, .0023, .0018, .0017] % Parameter not set Ohm  tau4_mat=[20, 36, 39; 31, 45, 39; 109, 105, 61; 36, 29, 26; 59, 77, 67; 40, 33, 29; 25, 39, 33] % Parameter not set s  tau4_vec=[36, 45, 105, 29, 77, 33, 39] % Parameter not set s  R5_mat=[.0109, .0029, .0013; .0069, .0024, .0012; .0047, .0026, .0013; .0034, .0016, .001; .0033, .0023, .0014; .0033, .0018, .0011; .0028, .0017, .0011] % Parameter not set Ohm  R5_vec=[.0029, .0024, .0026, .0016, .0023, .0018, .0017] % Parameter not set Ohm  tau5_mat=[20, 36, 39; 31, 45, 39; 109, 105, 61; 36, 29, 26; 59, 77, 67; 40, 33, 29; 25, 39, 33] % Parameter not set s  tau5_vec=[36, 45, 105, 29, 77, 33, 39] % Parameter not set s  prm_fade=simscape.enum.tablebattery.prm_fade.tableN  N0=100 % Parameter not set  dV0=0 % Parameter not set  dR0=0 % Parameter not set  dAH=0 % Parameter not set  dRleak=0 % Parameter not set  dR1=0 % Parameter not set  dR2=0 % Parameter not set  dR3=0 % Parameter not set  dR4=0 % Parameter not set  dR5=0 % Parameter not set  N0vec=[0 49 97 145 193 241 289 337 385 433 481 529 577 625 673 721 769 817 865 913 961 1009 1057 1105 1153 1201 1249 1297 1345 1393 1441 1489 1537 1585 1633 1681 1729 1777 1825 1873 1921 1969 2017 2065 2113 2161 2209 2257 2305 2353 2401 2449 2497 2545 2593 2641 2689 2737 2785 2833 2881 2929 2977 3025 3073 3121 3169 3217 3265 3313 3361 3409 3457 3505 3553 3601 3649 3697 3745 3793 3841 3889 3937 3985 4033 4081 4129 4177 4225 4273 4321 4369 4417 4465 4513 4561 4609 4657 4705 4753] % Datasheet derived  Tfadevec=[298.15, 323.15] % Parameter not set K  dV0vec=[0 -0.3454 -0.6908 -0.9359 -1.1676 -1.2672 -1.3271 -1.3712 -1.3796 -1.388 -1.3952 -1.402 -1.4086 -1.4146 -1.4207 -1.4251 -1.4284 -1.4315 -1.4266 -1.421 -1.4155 -1.4126 -1.4098 -1.4073 -1.4101 -1.4131 -1.4208 -1.4293 -1.4381 -1.447 -1.458 -1.4708 -1.4792 -1.4819 -1.4846 -1.4851 -1.4846 -1.4841 -1.4836 -1.483 -1.4824 -1.4819 -1.4816 -1.4821 -1.4826 -1.4864 -1.4903 -1.4956 -1.5014 -1.5097 -1.5201 -1.5313 -1.5437 -1.5564 -1.5697 -1.5877 -1.609 -1.6303 -1.6517 -1.6733 -1.6925 -1.7109 -1.7294 -1.7531 -1.7804 -1.8107 -1.8457 -1.8808 -1.9156 -1.9505 -1.9835 -2.0164 -2.048 -2.0852 -2.1232 -2.1613 -2.1969 -2.2314 -2.2586 -2.2847 -2.3081 -2.3315 -2.3541 -2.3775 -2.4018 -2.4263 -2.4508 -2.4714 -2.4903 -2.5029 -2.5135 -2.5281 -2.5444 -2.5606 -2.5769 -2.589 -2.5984 -2.6056 -2.6113 -2.617] % Datasheet derived  dR0vec=[0 0 0 0 0 0 0 0 0 0 0 0 0 0 0 0 0 0 0 0 0 0 0 0 0 0 0 0 0 0 0 0 0 0 0 0 0 0 0 0 0 0 0 0 0 0 0 0 0 0 0 0 0 0 0 0 0 0 0 0 0 0 0 0 0 0 0 0 0 0 0 0 0 0 0 0 0 0 0 0 0 0 0 0 0 0 0 0 0 0 0 0 0 0 0 0 0 0 0 0] % Parameter assumed  dAHvec=[0 -0.472 -0.944 -1.416 -1.889 -2.306 -2.716 -3.125 -3.535 -3.944 -4.342 -4.723 -5.104 -5.485 -5.867 -6.248 -6.629 -6.972 -7.314 -7.656 -7.997 -8.339 -8.681 -9.022 -9.457 -9.923 -10.389 -10.855 -11.321 -11.787 -12.254 -12.72 -13.106 -13.491 -13.876 -14.262 -14.647 -15.032 -15.417 -15.837 -16.264 -16.69 -17.116 -17.542 -17.987 -18.438 -18.889 -19.341 -19.792 -20.243 -20.694 -21.177 -21.71 -22.243 -22.776 -23.309 -23.842 -24.376 -24.909 -25.442 -25.915 -26.366 -26.816 -27.266 -27.717 -28.167 -28.617 -29.068 -29.518 -29.968 -30.419 -30.869 -31.319 -31.858 -32.41 -32.961 -33.512 -34.063 -34.615 -35.166 -35.717 -36.269 -36.802 -37.314 -37.826 -38.339 -38.851 -39.363 -39.875 -40.388 -40.9 -41.603 -42.38 -43.158 -43.935 -44.712 -45.49 -46.267 -47.044 -47.822] % Datasheet derived  dRleakvec=[0, 0, 0, 0] % Parameter not set  dR1vec=[0, 0, 0, 0] % Parameter not set  dR2vec=[0, 0, 0, 0] % Parameter not set  dR3vec=[0, 0, 0, 0] % Parameter not set  dR4vec=[0, 0, 0, 0] % Parameter not set  dR5vec=[0, 0, 0, 0] % Parameter not set  dV0mat=[0, 0; 0, 0; 0, 0; 0, 0] % Parameter not set  dR0mat=[0, 0; 0, 0; 0, 0; 0, 0] % Parameter not set  dAHmat=[0, 0; 0, 0; 0, 0; 0, 0] % Parameter not set  dRleakmat=[0, 0; 0, 0; 0, 0; 0, 0] % Parameter not set  dR1mat=[0, 0; 0, 0; 0, 0; 0, 0] % Parameter not set  dR2mat=[0, 0; 0, 0; 0, 0; 0, 0] % Parameter not set  dR3mat=[0, 0; 0, 0; 0, 0; 0, 0] % Parameter not set  dR4mat=[0, 0; 0, 0; 0, 0; 0, 0] % Parameter not set  dR5mat=[0, 0; 0, 0; 0, 0; 0, 0] % Parameter not set  prm_age_modeling=simscape.enum.tablebattery.prm_age_modeling.equation  storage_dt_age_vec=[0] % Parameter not set d  storage_T_age_vec=[273] % Parameter not set K  prm_age_OCV=simscape.enum.tablebattery.prm_age_OCV.OCV  OCV_age=0.9 % Parameter not set  SOC_age=0.6 % Parameter not set  prm_age_resistance=simscape.enum.tablebattery.prm_age.disabled  OCV_scaling_age_resistance=2.2134e6 % Parameter not set  OCV_offset_age_resistance=1.632e6 % Parameter not set  temp_exp_age_resistance=0.515833569 % Parameter not set V  t_exp_age_resistance=0.75 % Parameter not set  T_age_vec_resistance=[273.15, 298.15, 323.15] % Parameter not set K  dt_age_vec_resistance=[0, 90, 180, 270] % Parameter not set d  dR0_age_vec=[0, 0, 0] % Parameter not set  t_meas_dR0_age=100 % Parameter not set d  dR0_age_mat=[0, 0, 0; 0, 0, 0; 0, 0, 0; 0, 0, 0] % Parameter not set  prm_age_capacity=simscape.enum.tablebattery.prm_age.disabled  OCV_scaling_age_capacity=1.5097e07 % Parameter not set  OCV_offset_age_capacity=8.3625e06 % Parameter not set  temp_exp_age_capacity=0.6011 % Parameter not set V  t_exp_age_capacity=0.75 % Parameter not set  T_age_vec_capacity=[273.15, 298.15, 323.15] % Parameter not set K  dt_age_vec_capacity=[0, 90, 180, 270] % Parameter not set d  dAH_age_vec=[0, 0, 0] % Parameter not set  t_meas_dAH_age=100 % Parameter not set d  dAH_age_mat=[0, 0, 0; 0, 0, 0; 0, 0, 0; 0, 0, 0] % Parameter not set  thermal_port=simscape.enum.thermaleffects.model  temperature=298.15 % Parameter not set K  thermal_mass=16830 % Parameter assumed J/K  i_specify=off  i_priority=None  i=0 A  i_nominal_specify=off  i_nominal_value=1  i_nominal_unit=A  v_specify=off  v_priority=None  v=0 V  v_nominal_specify=off  v_nominal_value=1  v_nominal_unit=V  stateOfCharge_specify=off  stateOfCharge_priority=High  stateOfCharge=1  stateOfCharge_nominal_specify=off  stateOfCharge_nominal_value=1  stateOfCharge_nominal_unit=1  num_cycles_specify=off  num_cycles_priority=High  num_cycles=0  num_cycles_nominal_specify=off  num_cycles_nominal_value=1  num_cycles_nominal_unit=1  cell_temperature_specify=off  cell_temperature_priority=High  cell_temperature=298.15 K  cell_temperature_nominal_specify=off  cell_temperature_nominal_value=1  cell_temperature_nominal_unit=K
      settings: AttributesFormatString=Valence:U27_36XP
      settings: LibrarySourceBlock=|
      | batt_lib/Cells/Battery
      | (Table-Based)
  Capacity (Ah) : Gain  Gain=BatteryCap/1000
  Constant : Constant  Value=EngPowSL
  Constant1 : Constant  Value=0
  Controlled Current Source1 : fl_lib/Electrical/Electrical Sources/Controlled Current Source
  Convective Heat Transfer : fl_lib/Thermal/Thermal Elements/Convective Heat Transfer  thermal_type=foundation.enum.constant_variable.constant  area=1e-4 m^2  heat_tr_coeff=20 W/(K*m^2)  min_heat_tr_coeff=1e-3 W/(K*m^2)  T_specify=off  T_priority=None  T=0 K  T_nominal_specify=off  T_nominal_value=1  T_nominal_unit=K  Q_specify=off  Q_priority=None  Q=0 W  Q_nominal_specify=off  Q_nominal_value=1  Q_nominal_unit=W
  Discharge Rate : Constant  Value=BatteryDischrgRate
  Display3 : Display
  Display4 : Display
  Display5 : Display
  Divide1 : Product  Inputs=*/
  Electrical Reference : fl_lib/Electrical/Electrical Elements/Electrical Reference
  Excess Power : Display
  Gain : Gain  Gain=Preq2RPM
  Gain1 : Gain  Gain=1/1.225
  Gain3 : Gain  Gain=RPM2Vreq
  Gain4 : Gain  Gain=1000
  Minus2 : Sum  Inputs=-+
  Motor RPM : Display
  Old Battery Models : Subsystem  Commented=on
  PS-Simulink Converter : nesl_utility/PS-Simulink Converter  PhysicalDomain=network_engine_domain  SubClassName=ps_output  LeftPortType=input  RightPortType=output  PseudoPeriodic=off  Frequencies=[]  VectorFormat=inherit  Unit=inherit  AffineConversion=off
  PS-Simulink Converter1 : nesl_utility/PS-Simulink Converter  PhysicalDomain=network_engine_domain  SubClassName=ps_output  LeftPortType=input  RightPortType=output  PseudoPeriodic=off  Frequencies=[]  VectorFormat=inherit  Unit=inherit  AffineConversion=off
  PS-Simulink Converter2 : nesl_utility/PS-Simulink Converter  PhysicalDomain=network_engine_domain  SubClassName=ps_output  LeftPortType=input  RightPortType=output  PseudoPeriodic=off  Frequencies=[]  VectorFormat=inherit  Unit=inherit  AffineConversion=off
  Product : Product
  Saturation Dynamic : simulink/Discontinuities/Saturation Dynamic  OutMin=[]  OutMax=[]  OutDataTypeStr=Inherit: Same as second input  OutDataType=fixdt(1, 16)  OutScaling=2^-10  DoSatur=off
  Simulink-PS Converter : nesl_utility/Simulink-PS Converter  PhysicalDomain=network_engine_domain  SubClassName=ps_input  LeftPortType=input  RightPortType=output  PseudoPeriodic=off  Frequencies=[]  NoiseDistribution=none  NoiseParameters=[]  Unit=1  AffineConversion=off  FilteringAndDerivatives=provide  SimscapeFilterOrder=1  InputFilterTimeConstant=0.001  UdotUserProvided=0
  Solver Configuration : nesl_utility/Solver Configuration  PhysicalDomain=network_engine_domain  SubClassName=solver  LeftPortType=input  RightPortType=generic  Tones=[]  Harmonics=[]  SimulateNoise=off  Profile=off  UseLocalSampling=off  EnableSwitchedLinearOptims=on  FrequencyDomain=off  UseCCode=off  RelTol=0.001  AbsTol=0.001  MinStep=1e-09  ToWorkspace=off  RevertToSquareIcSolve=off  NumHomotopyIterations=100  PhasorMode=off  PhasorModeNumHarmonics=1  ConsistencySolver=NEWTON_XTOL_AFTER_FTOL  IndexReductionMethod=DerivativeReplacement  DoDC=off  ResidualTolerance=1e-09  ConsistencyTolSource=GLOBAL  ConsistencyAbsTol=0.001  ConsistencyRelTol=0.001  ConsistencyTolFactor=0.001  UseLocalSolver=off  LocalSolverChoice=NE_BACKWARD_EULER_ADVANCER  ResolveIndetEquations=on  FunctionEvalNumThread=1  LocalSolverSampleTime=0.001  DoFixedCost=off  MaxNonlinIter=3  MaxModeIter=2  ComputeImpulses=off  ImpulseIterations=2  LinearAlgebra=auto  LinearAlgebraNumThread=0  EquationFormulation=NE_TIME_EF  DelaysMemoryBudget=1024  AutomaticFiltering=on  FilteringTimeConstant=0.001  PartitionStorageMethod=AS_NEEDED  PartitionMemoryBudget=1024  PartitionMethod=ROBUST  MultibodyUseLocalSolver=off  MultibodyLocalSolverChoice=ODE1  MultibodyLocalSolverSampleTime=0.001
  Temperature Sensor : fl_lib/Thermal/Thermal Sensors/Temperature Sensor  temperature_measure=foundation.enum.MeasurementReference.difference
  Temperature Source : fl_lib/Thermal/Thermal Sources/Temperature Source  temperature=293.15 K
  Thermal Reference : fl_lib/Thermal/Thermal Elements/Thermal Reference
  Voltage Sensor : fl_lib/Electrical/Electrical Sensors/Voltage Sensor
  Battery State : Outport
  wires:
  Constant/1 -> Product/1
  airdensity/1 -> Gain1/1
  Gain1/1 -> Product/2
  Product/1 -> Minus2/2
  Minus2/1 -> Excess Power/1
  Preq/1 -> Gain/1, Minus2/1, Gain4/1
  Gain4/1 -> Divide1/1
  Gain3/1 -> Divide1/2
  Divide1/1 -> Saturation Dynamic/2  "Areq"
  Gain/1 -> Motor RPM/1, Gain3/1
  Discharge Rate/1 -> Capacity (Ah)/1
  Capacity (Ah)/1 -> Saturation Dynamic/1
  Constant1/1 -> Saturation Dynamic/3
  PS-Simulink Converter2/1 -> Battery State/1, Display4/1
  PS-Simulink Converter1/1 -> Display3/1
  PS-Simulink Converter/1 -> Display5/1
  Saturation Dynamic/1 -> Simulink-PS Converter/1
  connections:
  Voltage Sensor/LConn1 -- Battery (Table-Based)/LConn1 -- Controlled Current Source1/RConn2
  Battery (Table-Based)/RConn2 -- Convective Heat Transfer/LConn1 -- Temperature Sensor/LConn1
  Battery (Table-Based)/RConn1 -- Voltage Sensor/RConn2 -- Controlled Current Source1/LConn1 -- Electrical Reference/LConn1 -- Solver Configuration/RConn1
  PS-Simulink Converter2/LConn1 -- Battery (Table-Based)/LConn2
  Temperature Source/LConn1 -- Convective Heat Transfer/RConn1
  Simulink-PS Converter/RConn1 -- Controlled Current Source1/RConn1
  Temperature Sensor/RConn2 -- PS-Simulink Converter/LConn1
  Thermal Reference/LConn1 -- Temperature Sensor/RConn1
  PS-Simulink Converter1/LConn1 -- Voltage Sensor/RConn1

== system HeliDraft_26_02_2025/Helicopter Model/Forces and Moments/Fuselage ==
  rho : Inport
  Product : Product
  Out1 : Outport
  Out2 : Outport  Port=2
  Pparasite : Outport  Port=3

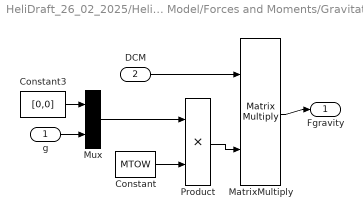
== system HeliDraft_26_02_2025/Helicopter Model/Forces and Moments/Gravitational ==
  g : Inport
  DCM : Inport  Port=2
  Constant : Constant  Value=MTOW
  Constant3 : Constant  Value=[0,0]
  MatrixMultiply : Product  Multiplication=Matrix(*)
  Mux : Mux  Inputs=2
  Product : Product
  Fgravity : Outport
  wires:
  DCM/1 -> MatrixMultiply/1
  MatrixMultiply/1 -> Fgravity/1
  Product/1 -> MatrixMultiply/2
  g/1 -> Mux/2
  Constant/1 -> Product/2
  Mux/1 -> Product/1
  Constant3/1 -> Mux/1

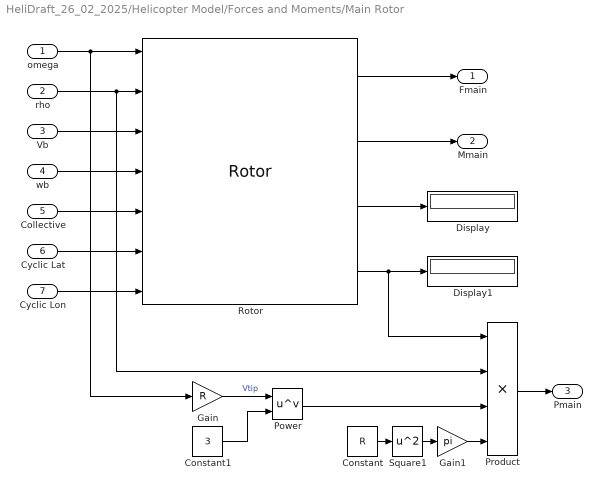
== system HeliDraft_26_02_2025/Helicopter Model/Forces and Moments/Main Rotor ==
  omega : Inport
  rho : Inport  Port=2
  Vb : Inport  Port=3
  wb : Inport  Port=4
  Collective : Inport  Port=5
  Cyclic Lat : Inport  Port=6
  Cyclic Lon : Inport  Port=7
  Constant : Constant  Value=R
  Constant1 : Constant  Value=3
  Display : Display
  Display1 : Display
  Gain : Gain  Gain=R
  Gain1 : Gain  Gain=pi
  Power : Math  Operator=pow
  Product : Product  Inputs=4
  Rotor : Rotor  modelMode=With flap effects  controlInput=on  CTCQMode=Compute using BEMT  Nb=Nb  CTout=on  radius=R  chord=c  clalpha=CLalpha  cd0=0.009  gamma=10  thetaRoot=BldRootAng  thetaTwist=BldTwstAng
  Square1 : Math  Operator=square
  Fmain : Outport
  Mmain : Outport  Port=2
  Pmain : Outport  Port=3
  wires:
  omega/1 -> Rotor/1, Gain/1
  Rotor/1 -> Fmain/1
  rho/1 -> Rotor/2, Product/2
  Rotor/2 -> Mmain/1
  Collective/1 -> Rotor/5
  Rotor/3 -> Display/1
  Rotor/4 -> Product/1, Display1/1
  Cyclic Lon/1 -> Rotor/7
  Cyclic Lat/1 -> Rotor/6
  Vb/1 -> Rotor/3
  wb/1 -> Rotor/4
  Power/1 -> Product/3
  Gain/1 -> Power/1  "Vtip"
  Constant/1 -> Square1/1
  Square1/1 -> Gain1/1
  Gain1/1 -> Product/4
  Constant1/1 -> Power/2
  Product/1 -> Pmain/1
